simulink model "System23a"  (R2023a)
settings: Solver=ode23t  StartTime=0.0  StopTime=100  MaxStep=0.005  RelTol=1e-3
settings Model: Creator=andriyanov_ilya  LastModifiedBy=user

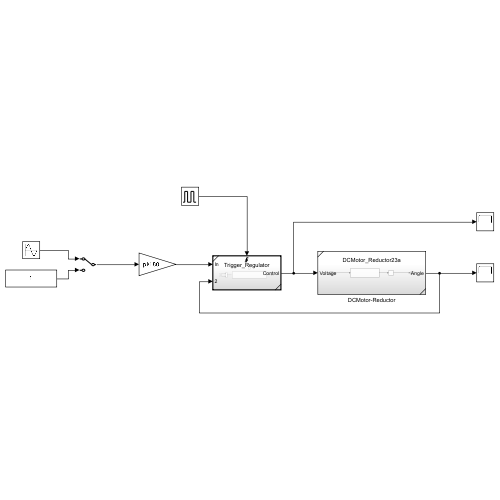
[thumbnail: Simulink's stored preview of the top-level diagram]
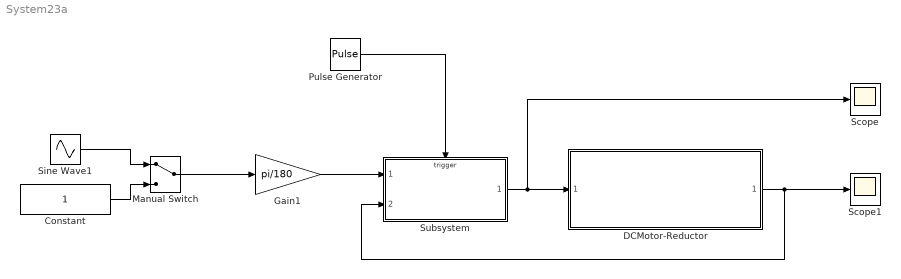
== system System23a ==
  Constant : Constant
  DCMotor-Reductor : Subsystem  ReferencedSubsystem=DCMotor_Reductor23a
  Gain1 : Gain  Gain=pi/180
  Manual Switch : ManualSwitch
  Pulse Generator : DiscretePulseGenerator  PulseType=Time based  Period=0.005  PulseWidth=5
  Scope : Scope
  Scope1 : Scope
  Sine Wave1 : Sin  Amplitude=140  Frequency=0.63  SampleTime=0
  Subsystem : Subsystem  ReferencedSubsystem=Trigger_Regulator
  wires:
  DCMotor-Reductor/1 -> Scope1/1, Subsystem/2
  Constant/1 -> Manual Switch/2
  Sine Wave1/1 -> Manual Switch/1
  Manual Switch/1 -> Gain1/1
  Gain1/1 -> Subsystem/1
  Subsystem/1 -> Scope/1, DCMotor-Reductor/1
  Pulse Generator/1 -> Subsystem/Trigger
